simulink subsystem "Bluetooth_Datos"  (R2024b)
settings: Solver=VariableStepAuto  StartTime=0.0  StopTime=10.0  RelTol=1e-3
libraries: simulink x16, arduinolib x1
settings Model: Creator=Chenfu  LastModifiedBy=Chenfu

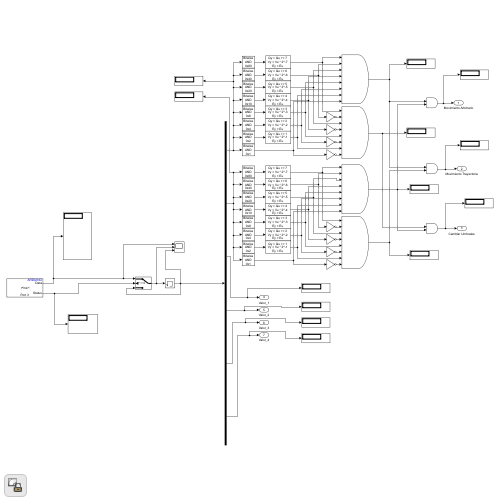
[thumbnail: Simulink's stored preview of the top-level diagram]
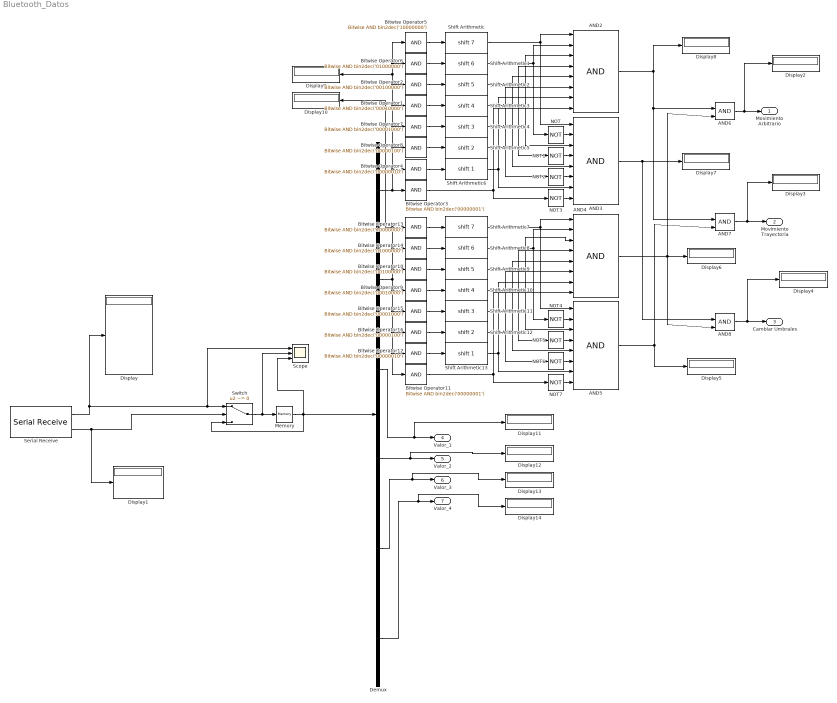
== system Bluetooth_Datos ==
  AND{2..5} (4 alike) : Logic  Inputs=8  IconShape=distinctive  AllPortsSameDT=off  OutDataTypeStr=boolean
  AND6 : Logic  IconShape=distinctive  AllPortsSameDT=off  OutDataTypeStr=boolean
  AND7 : Logic  IconShape=distinctive  AllPortsSameDT=off  OutDataTypeStr=boolean
  AND8 : Logic  IconShape=distinctive  AllPortsSameDT=off  OutDataTypeStr=boolean
  Bitwise Operator1 : simulink/Logic and Bit Operations/Bitwise Operator  logicop=AND  UseBitMask=on  BitMask=bin2dec('00010000')  BitMaskRealWorld=Stored Integer
  Bitwise Operator10 : simulink/Logic and Bit Operations/Bitwise Operator  logicop=AND  UseBitMask=on  BitMask=bin2dec('00100000')  BitMaskRealWorld=Stored Integer
  Bitwise Operator11 : simulink/Logic and Bit Operations/Bitwise Operator  logicop=AND  UseBitMask=on  BitMask=bin2dec('00000001')  BitMaskRealWorld=Stored Integer
  Bitwise Operator12 : simulink/Logic and Bit Operations/Bitwise Operator  logicop=AND  UseBitMask=on  BitMask=bin2dec('00000010')  BitMaskRealWorld=Stored Integer
  Bitwise Operator13 : simulink/Logic and Bit Operations/Bitwise Operator  logicop=AND  UseBitMask=on  BitMask=bin2dec('10000000')  BitMaskRealWorld=Stored Integer
  Bitwise Operator14 : simulink/Logic and Bit Operations/Bitwise Operator  logicop=AND  UseBitMask=on  BitMask=bin2dec('01000000')  BitMaskRealWorld=Stored Integer
  Bitwise Operator15 : simulink/Logic and Bit Operations/Bitwise Operator  logicop=AND  UseBitMask=on  BitMask=bin2dec('00001000')  BitMaskRealWorld=Stored Integer
  Bitwise Operator16 : simulink/Logic and Bit Operations/Bitwise Operator  logicop=AND  UseBitMask=on  BitMask=bin2dec('00000100')  BitMaskRealWorld=Stored Integer
  Bitwise Operator2 : simulink/Logic and Bit Operations/Bitwise Operator  logicop=AND  UseBitMask=on  BitMask=bin2dec('00100000')  BitMaskRealWorld=Stored Integer
  Bitwise Operator3 : simulink/Logic and Bit Operations/Bitwise Operator  logicop=AND  UseBitMask=on  BitMask=bin2dec('00000001')  BitMaskRealWorld=Stored Integer
  Bitwise Operator4 : simulink/Logic and Bit Operations/Bitwise Operator  logicop=AND  UseBitMask=on  BitMask=bin2dec('00000010')  BitMaskRealWorld=Stored Integer
  Bitwise Operator5 : simulink/Logic and Bit Operations/Bitwise Operator  logicop=AND  UseBitMask=on  BitMask=bin2dec('10000000')  BitMaskRealWorld=Stored Integer
  Bitwise Operator6 : simulink/Logic and Bit Operations/Bitwise Operator  logicop=AND  UseBitMask=on  BitMask=bin2dec('01000000')  BitMaskRealWorld=Stored Integer
  Bitwise Operator7 : simulink/Logic and Bit Operations/Bitwise Operator  logicop=AND  UseBitMask=on  BitMask=bin2dec('00001000')  BitMaskRealWorld=Stored Integer
  Bitwise Operator8 : simulink/Logic and Bit Operations/Bitwise Operator  logicop=AND  UseBitMask=on  BitMask=bin2dec('00000100')  BitMaskRealWorld=Stored Integer
  Bitwise Operator9 : simulink/Logic and Bit Operations/Bitwise Operator  logicop=AND  UseBitMask=on  BitMask=bin2dec('00010000')  BitMaskRealWorld=Stored Integer
  Demux : Demux  Outputs=6
  Display{,1..14} (15 alike) : Display
  Memory : Memory
  NOT{,1..7} (8 alike) : Logic  Operator=NOT  IconShape=distinctive  AllPortsSameDT=off  OutDataTypeStr=boolean
  Scope : Scope  NumInputPorts=3
  Serial Receive : arduinolib/Serial Receive  portNumber=3  DataType=uint8  blockPlatform=ARDUINO  TimeOut=0  MaxDataLength=10  isARMArch=off  DataLengthOption=Length via dialog  Datalength=6  Header=[]  Terminator=[]  SampleTime=0.1  ShowOutStatus=on
  Shift Arithmetic : ArithShift  BitShiftNumber=7
  Shift Arithmetic1 : ArithShift  BitShiftNumber=6
  Shift Arithmetic10 : ArithShift  BitShiftNumber=4
  Shift Arithmetic11 : ArithShift  BitShiftNumber=3
  Shift Arithmetic12 : ArithShift  BitShiftNumber=2
  Shift Arithmetic13 : ArithShift  BitShiftNumber=1
  Shift Arithmetic2 : ArithShift  BitShiftNumber=5
  Shift Arithmetic3 : ArithShift  BitShiftNumber=4
  Shift Arithmetic4 : ArithShift  BitShiftNumber=3
  Shift Arithmetic5 : ArithShift  BitShiftNumber=2
  Shift Arithmetic6 : ArithShift  BitShiftNumber=1
  Shift Arithmetic7 : ArithShift  BitShiftNumber=7
  Shift Arithmetic8 : ArithShift  BitShiftNumber=6
  Shift Arithmetic9 : ArithShift  BitShiftNumber=5
  Switch : Switch  Criteria=u2 ~= 0  SaturateOnIntegerOverflow=off  InputSameDT=off
  Movimiento Arbitrario : Outport
  Movimiento Trayectoria : Outport  Port=2
  Cambiar Umbrales : Outport  Port=3
  Valor_1 : Outport  Port=4
  Valor_2 : Outport  Port=5
  Valor_3 : Outport  Port=6
  Valor_4 : Outport  Port=7
  wires:
  Serial Receive/1 -> Switch/1, Scope/1, Display/1
  Switch/1 -> Memory/1, Scope/2
  Memory/1 -> Demux/1, Switch/3, Scope/3
  Serial Receive/2 -> Switch/2, Display1/1
  Demux/6 -> Valor_4/1, Display14/1
  Demux/5 -> Valor_3/1, Display13/1
  Demux/4 -> Valor_2/1, Display12/1
  Demux/3 -> Valor_1/1, Display11/1
  AND8/1 -> Cambiar Umbrales/1, Display4/1
  AND7/1 -> Movimiento Trayectoria/1, Display3/1
  AND6/1 -> Movimiento Arbitrario/1, Display2/1
  AND3/1 -> AND8/1, Display7/1
  AND5/1 -> AND7/2, Display5/1
  AND4/1 -> AND8/2, AND6/2, Display6/1
  AND2/1 -> AND6/1, AND7/1, Display8/1
  Demux/2 -> Bitwise Operator9/1, Bitwise Operator16/1, Bitwise Operator12/1, Bitwise Operator11/1, Bitwise Operator15/1, Bitwise Operator10/1, Bitwise Operator14/1, Bitwise Operator13/1, Display10/1
  Shift Arithmetic13/1 -> AND4/7, AND5/7
  Bitwise Operator16/1 -> Shift Arithmetic12/1
  Bitwise Operator9/1 -> Shift Arithmetic10/1
  Bitwise Operator15/1 -> Shift Arithmetic11/1
  Bitwise Operator13/1 -> Shift Arithmetic7/1
  NOT7/1 -> AND5/8
  Shift Arithmetic8/1 -> AND4/2, NOT4/1
  Shift Arithmetic9/1 -> AND5/3, AND4/3
  Bitwise Operator10/1 -> Shift Arithmetic9/1
  Bitwise Operator11/1 -> AND4/8, NOT7/1
  Bitwise Operator12/1 -> Shift Arithmetic13/1
  Shift Arithmetic11/1 -> AND4/5, AND5/5
  Shift Arithmetic10/1 -> NOT5/1, AND4/4
  Shift Arithmetic7/1 -> AND4/1, AND5/1
  Bitwise Operator14/1 -> Shift Arithmetic8/1
  NOT6/1 -> AND5/6
  NOT4/1 -> AND5/2
  NOT5/1 -> AND5/4
  Shift Arithmetic12/1 -> AND4/6, NOT6/1
  Shift Arithmetic/1 -> AND2/1, AND3/1
  Shift Arithmetic1/1 -> AND2/2, NOT/1
  Shift Arithmetic2/1 -> AND3/3, AND2/3
  Shift Arithmetic3/1 -> NOT1/1, AND2/4
  Shift Arithmetic4/1 -> AND2/5, AND3/5
  Shift Arithmetic5/1 -> AND2/6, NOT2/1
  Shift Arithmetic6/1 -> AND2/7, AND3/7
  Bitwise Operator3/1 -> AND2/8, NOT3/1
  NOT3/1 -> AND3/8
  NOT2/1 -> AND3/6
  NOT1/1 -> AND3/4
  NOT/1 -> AND3/2
  Bitwise Operator5/1 -> Shift Arithmetic/1
  Bitwise Operator6/1 -> Shift Arithmetic1/1
  Bitwise Operator2/1 -> Shift Arithmetic2/1
  Bitwise Operator1/1 -> Shift Arithmetic3/1
  Bitwise Operator7/1 -> Shift Arithmetic4/1
  Bitwise Operator8/1 -> Shift Arithmetic5/1
  Bitwise Operator4/1 -> Shift Arithmetic6/1
  Demux/1 -> Bitwise Operator3/1, Bitwise Operator4/1, Bitwise Operator8/1, Bitwise Operator7/1, Bitwise Operator1/1, Bitwise Operator2/1, Bitwise Operator6/1, Bitwise Operator5/1, Display9/1
